simulink model "BE_simu4"  (R2018b)
settings: Solver=VariableStepAuto  StartTime=0.0  StopTime=100  RelTol=1e-3
values from neighbouring files (symbols this model uses):
  assist = 2    [BE_eletr.m]
  Jt = M*Rw^2    (= 10.0188)    [BE_eletr.m]
  lambm = 0.0744    [BE_eletr.m]
  Ls = 0.0021    [BE_eletr.m]
  Np = 52    [BE_eletr.m]
  Rpp = 36/16    (= 2.25)    [BE_eletr.m]
  Rs = 0.124    [BE_eletr.m]
  s = 0.07    [BE_eletr.m]
libraries: simulink x2
settings Model: Creator=antoi  LastModifiedBy=piffercg
settings DataIOCC: ReturnWorkspaceOutputs=on
settings DebuggingCC: AlgebraicLoopMsg=none

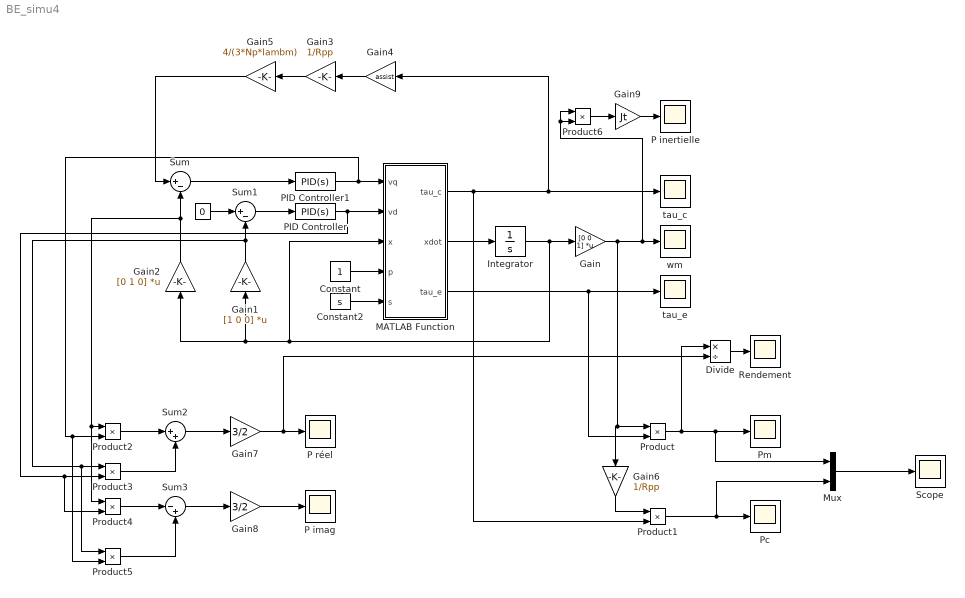
== system BE_simu4 ==
  " " : Constant  Value=0
  Constant : Constant
  Constant2 : Constant  Value=s
  Divide : Product  Inputs=*/
  Gain : Gain  Gain=[0 0 1]  Multiplication=Matrix(K*u)
  Gain1 : Gain  Gain=[1 0 0]  Multiplication=Matrix(K*u)
  Gain2 : Gain  Gain=[0 1 0]  Multiplication=Matrix(K*u)
  Gain3 : Gain  Gain=1/Rpp
  Gain4 : Gain  Gain=assist
  Gain5 : Gain  Gain=4/(3*Np*lambm)
  Gain6 : Gain  Gain=1/Rpp
  Gain7 : Gain  Gain=3/2
  Gain8 : Gain  Gain=3/2
  Gain9 : Gain  Gain=Jt
  Integrator : Integrator  InitialCondition=[0 ;0 ;0]
  MATLAB Function : MATLAB Function  TreatAsAtomicUnit=on
  Mux : Mux  Inputs=2
  "P imag " : Scope
  P inertielle : Scope
  "P réel " : Scope
  PID Controller : simulink/Continuous/PID Controller  Controller=PID  Form=Parallel  TimeDomain=Continuous-time  SampleTime=-1  IntegratorMethod=Forward Euler  FilterMethod=Forward Euler  ControllerParametersSource=internal  P=Rs  I=Rs*Rs/Ls  D=0  UseFilter=on  N=100  TunerSelectOption=Transfer Function Based (PID Tuner App)  InitialConditionSource=internal  InitialConditionForIntegrator=0  InitialConditionForFilter=0  DifferentiatorICPrevScaledInput=0  ExternalReset=none  TrackingMode=off  Kt=1  LimitOutput=off  UpperSaturationLimit=inf  LowerSaturationLimit=-inf  LinearizeAsGain=on  AntiWindupMode=none  Kb=1  POutMin=[]  POutMax=[]  IOutMin=[]  IOutMax=[]  DOutMin=[]  DOutMax=[]  NOutMin=[]  NOutMax=[]  SumOutMin=[]  SumOutMax=[]  SaturationOutMin=[]  SaturationOutMax=[]  PParamMin=[]  PParamMax=[]  IParamMin=[]  IParamMax=[]  DParamMin=[]  DParamMax=[]  NParamMin=[]  NParamMax=[]  KbParamMin=[]  KbParamMax=[]  KtParamMin=[]  KtParamMax=[]  KbOutMin=[]  KbOutMax=[]  KtOutMin=[]  KtOutMax=[]  IntegratorOutMin=[]  IntegratorOutMax=[]  FilterOutMin=[]  FilterOutMax=[]  SumI1OutMin=[]  SumI1OutMax=[]  SumI2OutMin=[]  SumI2OutMax=[]  SumI3OutMin=[]  SumI3OutMax=[]  SumI4OutMin=[]  SumI4OutMax=[]  SumDOutMin=[]  SumDOutMax=[]  DifferentiatorOutMin=[]  DifferentiatorOutMax=[]  FilterDiffOutCoefMin=[]  FilterDiffOutCoefMax=[]  ReciprocalOutMin=[]  ReciprocalOutMax=[]  SumDenOutMin=[]  SumDenOutMax=[]  SumNumOutMin=[]  SumNumOutMax=[]  DivideOutMin=[]  DivideOutMax=[]  IntegratorContinuousStateAttributes=''  IntegratorStateMustResolveToSignalObject=off  IntegratorRTWStateStorageClass=Auto  FilterContinuousStateAttributes=''  FilterStateMustResolveToSignalObject=off  FilterRTWStateStorageClass=Auto  ParallelPVariant=InternalParameters  IdealPVariant=Disabled  IVariant=InternalParameters  DVariant=InternalParameters  IntegratorVariant=Continuous  SatVariant=Disabled  AWVariant=Passthrough  PCopyVariant=Disabled  TRVariant=Disabled  FdbkBlocksVariant=Forward  IdealPFdbkVariant=Disabled  SatFdbkVariant=Disabled  DerivativeFilterVariant=ContFilter  NVariant=InternalParameters  NCopyVariant=Disabled  FilterICVariant=InternalICsFilter  IntegratorICVariant=InternalICs  ExternalResetVariant=Disabled  TRSumVariant=Passthrough  SumFdbkVariant=Disabled  SumVariant=Sum_PID
  PID Controller1 : simulink/Continuous/PID Controller  Controller=PID  Form=Parallel  TimeDomain=Continuous-time  SampleTime=-1  IntegratorMethod=Forward Euler  FilterMethod=Forward Euler  ControllerParametersSource=internal  P=Rs  I=Rs*Rs/Ls  D=0  UseFilter=on  N=100  TunerSelectOption=Transfer Function Based (PID Tuner App)  InitialConditionSource=internal  InitialConditionForIntegrator=0  InitialConditionForFilter=0  DifferentiatorICPrevScaledInput=0  ExternalReset=none  TrackingMode=off  Kt=1  LimitOutput=off  UpperSaturationLimit=inf  LowerSaturationLimit=-inf  LinearizeAsGain=on  AntiWindupMode=none  Kb=1  POutMin=[]  POutMax=[]  IOutMin=[]  IOutMax=[]  DOutMin=[]  DOutMax=[]  NOutMin=[]  NOutMax=[]  SumOutMin=[]  SumOutMax=[]  SaturationOutMin=[]  SaturationOutMax=[]  PParamMin=[]  PParamMax=[]  IParamMin=[]  IParamMax=[]  DParamMin=[]  DParamMax=[]  NParamMin=[]  NParamMax=[]  KbParamMin=[]  KbParamMax=[]  KtParamMin=[]  KtParamMax=[]  KbOutMin=[]  KbOutMax=[]  KtOutMin=[]  KtOutMax=[]  IntegratorOutMin=[]  IntegratorOutMax=[]  FilterOutMin=[]  FilterOutMax=[]  SumI1OutMin=[]  SumI1OutMax=[]  SumI2OutMin=[]  SumI2OutMax=[]  SumI3OutMin=[]  SumI3OutMax=[]  SumI4OutMin=[]  SumI4OutMax=[]  SumDOutMin=[]  SumDOutMax=[]  DifferentiatorOutMin=[]  DifferentiatorOutMax=[]  FilterDiffOutCoefMin=[]  FilterDiffOutCoefMax=[]  ReciprocalOutMin=[]  ReciprocalOutMax=[]  SumDenOutMin=[]  SumDenOutMax=[]  SumNumOutMin=[]  SumNumOutMax=[]  DivideOutMin=[]  DivideOutMax=[]  IntegratorContinuousStateAttributes=''  IntegratorStateMustResolveToSignalObject=off  IntegratorRTWStateStorageClass=Auto  FilterContinuousStateAttributes=''  FilterStateMustResolveToSignalObject=off  FilterRTWStateStorageClass=Auto  ParallelPVariant=InternalParameters  IdealPVariant=Disabled  IVariant=InternalParameters  DVariant=InternalParameters  IntegratorVariant=Continuous  SatVariant=Disabled  AWVariant=Passthrough  PCopyVariant=Disabled  TRVariant=Disabled  FdbkBlocksVariant=Forward  IdealPFdbkVariant=Disabled  SatFdbkVariant=Disabled  DerivativeFilterVariant=ContFilter  NVariant=InternalParameters  NCopyVariant=Disabled  FilterICVariant=InternalICsFilter  IntegratorICVariant=InternalICs  ExternalResetVariant=Disabled  TRSumVariant=Passthrough  SumFdbkVariant=Disabled  SumVariant=Sum_PID
  Pc : Scope
  "Pm " : Scope
  Product{,1..6} (7 alike) : Product
  Rendement : Scope
  Scope : Scope
  Sum : Sum  Inputs=|+-
  Sum1 : Sum  Inputs=|+-
  Sum2 : Sum  Inputs=|++
  Sum3 : Sum  Inputs=|-+
  tau_c : Scope
  tau_e : Scope
  wm : Scope
  wires:
  Integrator/1 -> Gain/1, Gain1/1, Gain2/1, MATLAB Function/3(x)
  MATLAB Function/2(xdot) -> Integrator/1
  " "/1 -> Sum1/1
  Sum1/1 -> PID Controller/1
  PID Controller/1 -> MATLAB Function/2(vd), Product4/2, Product3/2
  PID Controller1/1 -> Product5/2, Product2/2, MATLAB Function/1(vq)
  Sum/1 -> PID Controller1/1
  Gain1/1 -> Product5/1, Product3/1, Sum1/2
  Gain2/1 -> Product4/1, Product2/1, Sum/2
  Constant2/1 -> MATLAB Function/5(s)
  MATLAB Function/1(tau_c) -> Product1/2, Gain4/1, tau_c/1
  MATLAB Function/3(tau_e) -> Product/2, tau_e/1
  Constant/1 -> MATLAB Function/4(p)
  Gain3/1 -> Gain5/1
  Gain5/1 -> Sum/1
  Gain4/1 -> Gain3/1
  Product/1 -> Divide/1, Mux/1, "Pm "/1
  Product1/1 -> Mux/2, Pc/1
  Mux/1 -> Scope/1
  Gain6/1 -> Product1/1
  Gain/1 -> Product/1, Gain6/1, Product6/1, Product6/2, wm/1
  Gain7/1 -> Divide/2, "P réel "/1
  Sum2/1 -> Gain7/1
  Product2/1 -> Sum2/1
  Product3/1 -> Sum2/2
  Sum3/1 -> Gain8/1
  Gain8/1 -> "P imag "/1
  Product4/1 -> Sum3/1
  Product5/1 -> Sum3/2
  Divide/1 -> Rendement/1
  Product6/1 -> Gain9/1
  Gain9/1 -> P inertielle/1

== matlab function BE_simu4/MATLAB Function ==
  data: tau_c output; vq input; vd input; xdot output; x input; tau_e output; p input; s input
function [tau_c,xdot,tau_e]= fcn(vq,vd,x,p,s)
    Rs = 0.124 ;
    Ls = 0.0021 ;
    lambm = 0.0744 ;
    Np = 52 ;
    M = 92 ;
    Rw = 0.33 ;
    Jt = M*Rw*Rw ;
    Ca = 0.18 ;
    g = 9.81 ;
    Rpp = 36/16;
    
    tau_e = (3*Np*lambm/4) * x(2) ;
    tau_c = (60 - (60/(4*pi))*x(3)*(16/36))*p ; 
    tau_load = M*g*s*Rw + Ca*(Rw^3)*(x(3)^2) ;
    
    xdot1 =  -(Rs/Ls)*x(1) + (Np/2)*x(2)*x(3) + vd/Ls ;
    xdot2 = -(Rs/Ls)*x(2) - (Np/2)*x(1)*x(3) - (Np/2)*(lambm/Ls)*x(3) + vq/Ls ; 
    xdot3 = (1/Jt)*(tau_e - tau_load + tau_c*(1/Rpp))  ;
    xdot=[xdot1 ; xdot2 ; xdot3] ;
end
